simulink model "obserwator"  (R2021b)
settings: Solver=VariableStepAuto  StartTime=0.0  StopTime=8  RelTol=1e-3
values from neighbouring files (symbols this model uses):
  K = zeros(1, 3)    [stp01.m]
  L = acker(A_1', C_1', Po)    [stp01.m]
  start_x = [0 0 0]    [stp01.m]
  Tp = 0.5    [stp01.m]
undefined symbols (not defined in the file or in its folder): A_1, C_1
settings Model: Creator=USER  LastModifiedBy=USER

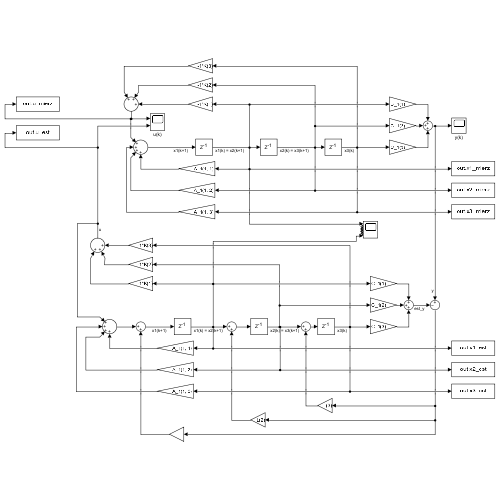
[thumbnail: Simulink's stored preview of the top-level diagram]
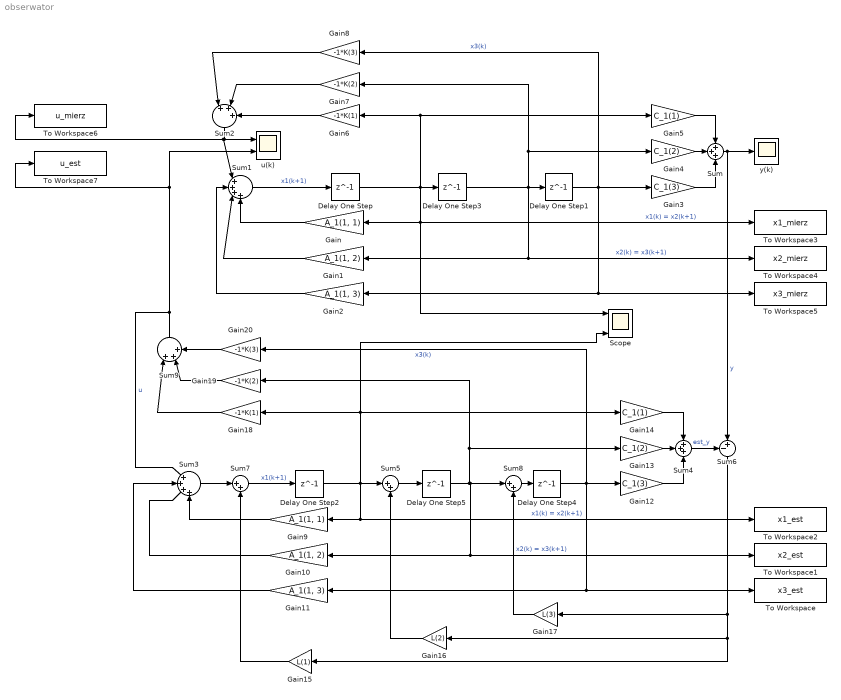
== system obserwator ==
  Delay One Step : Delay  DelayLength=1  InitialCondition=start_x(1)  SampleTime=Tp
  Delay One Step1 : Delay  DelayLength=1  InitialCondition=start_x(3)  SampleTime=Tp
  Delay One Step2 : Delay  DelayLength=1  InitialCondition=0  SampleTime=Tp
  Delay One Step3 : Delay  DelayLength=1  InitialCondition=start_x(2)  SampleTime=Tp
  Delay One Step4 : Delay  DelayLength=1  InitialCondition=0  SampleTime=Tp
  Delay One Step5 : Delay  DelayLength=1  InitialCondition=0  SampleTime=Tp
  Gain : Gain  Gain=A_1(1, 1)
  Gain1 : Gain  Gain=A_1(1, 2)
  Gain10 : Gain  Gain=A_1(1, 2)
  Gain11 : Gain  Gain=A_1(1, 3)
  Gain12 : Gain  Gain=C_1(3)
  Gain13 : Gain  Gain=C_1(2)
  Gain14 : Gain  Gain=C_1(1)
  Gain15 : Gain  Gain=L(1)
  Gain16 : Gain  Gain=L(2)
  Gain17 : Gain  Gain=L(3)
  Gain18 : Gain  Gain=-1*K(1)
  Gain19 : Gain  Gain=-1*K(2)
  Gain2 : Gain  Gain=A_1(1, 3)
  Gain20 : Gain  Gain=-1*K(3)
  Gain3 : Gain  Gain=C_1(3)
  Gain4 : Gain  Gain=C_1(2)
  Gain5 : Gain  Gain=C_1(1)
  Gain6 : Gain  Gain=-1*K(1)
  Gain7 : Gain  Gain=-1*K(2)
  Gain8 : Gain  Gain=-1*K(3)
  Gain9 : Gain  Gain=A_1(1, 1)
  Scope : Scope  NumInputPorts=6
  Sum : Sum  Inputs=+++
  Sum1 : Sum  Inputs=|++++
  Sum2 : Sum  Inputs=|+++
  Sum3 : Sum  Inputs=|++++
  Sum4 : Sum  Inputs=+++
  Sum5 : Sum  Inputs=|++
  Sum6 : Sum  Inputs=-+|
  Sum7 : Sum  Inputs=|++
  Sum8 : Sum  Inputs=|++
  Sum9 : Sum  Inputs=|+++
  To Workspace : ToWorkspace  VariableName=x3_est  SaveFormat=Structure With Time  SampleTime=Tp
  To Workspace1 : ToWorkspace  VariableName=x2_est  SaveFormat=Structure With Time  SampleTime=Tp
  To Workspace2 : ToWorkspace  VariableName=x1_est  SaveFormat=Structure With Time  SampleTime=Tp
  To Workspace3 : ToWorkspace  VariableName=x1_mierz  SaveFormat=Structure With Time  SampleTime=Tp
  To Workspace4 : ToWorkspace  VariableName=x2_mierz  SaveFormat=Structure With Time  SampleTime=Tp
  To Workspace5 : ToWorkspace  VariableName=x3_mierz  SaveFormat=Structure With Time  SampleTime=Tp
  To Workspace6 : ToWorkspace  VariableName=u_mierz  SaveFormat=Structure With Time  SampleTime=Tp
  To Workspace7 : ToWorkspace  VariableName=u_est  SaveFormat=Structure With Time  SampleTime=Tp
  u(k) : Scope  NumInputPorts=2
  y(k) : Scope
  wires:
  Sum2/1 -> Sum1/1, To Workspace6/1, u(k)/1
  Gain2/1 -> Sum1/2
  Gain5/1 -> Sum/1
  Delay One Step/1 -> Gain6/1, Gain5/1, Scope/1, To Workspace3/1, Gain/1, Delay One Step3/1  "x1(k) = x2(k+1)"
  Gain7/1 -> Sum2/2
  Gain8/1 -> Sum2/1
  Gain6/1 -> Sum2/3
  Delay One Step3/1 -> Gain7/1, Gain4/1, To Workspace4/1, Gain1/1, Delay One Step1/1  "x2(k) = x3(k+1)"
  Gain1/1 -> Sum1/3
  Gain3/1 -> Sum/3
  Sum1/1 -> Delay One Step/1  "x1(k+1)"
  Delay One Step1/1 -> Gain8/1, Gain3/1, To Workspace5/1, Gain2/1  "x3(k)"
  Sum/1 -> y(k)/1, Sum6/2  "y"
  Gain/1 -> Sum1/4
  Gain4/1 -> Sum/2
  Gain9/1 -> Sum3/4
  Delay One Step4/1 -> Gain20/1, Gain12/1, Gain11/1, To Workspace/1  "x3(k)"
  Gain10/1 -> Sum3/3
  Gain11/1 -> Sum3/2
  Gain13/1 -> Sum4/2
  Gain14/1 -> Sum4/1
  Gain12/1 -> Sum4/3
  Delay One Step2/1 -> Scope/6, Gain14/1, Gain18/1, Gain9/1, To Workspace2/1, Sum5/1  "x1(k) = x2(k+1)"
  Sum5/1 -> Delay One Step5/1
  Sum6/1 -> Gain15/1, Gain16/1, Gain17/1
  Sum4/1 -> Sum6/1  "est_y"
  Delay One Step5/1 -> Gain19/1, Gain13/1, To Workspace1/1, Gain10/1, Sum8/1  "x2(k) = x3(k+1)"
  Sum8/1 -> Delay One Step4/1
  Gain15/1 -> Sum7/2
  Gain17/1 -> Sum8/2
  Gain16/1 -> Sum5/2
  Gain20/1 -> Sum9/3
  Gain19/1 -> Sum9/2
  Gain18/1 -> Sum9/1
  Sum9/1 -> To Workspace7/1, u(k)/2, Sum3/1  "u"
  Sum7/1 -> Delay One Step2/1  "x1(k+1)"
  Sum3/1 -> Sum7/1
